simulink model "SF035A_DampgPahFwl"  (R2013b)
settings: Solver=FixedStepDiscrete  SolverMode=SingleTasking  StartTime=0.0  StopTime=1  FixedStep=0.002  RelTol=1e-3
undefined symbols (not defined in the file): ARCHGLBPRM_2MILLISEC_SEC_F32, DampgPahFwlDampgCmdFwlOverLimDiagcFailStep, DampgPahFwlDampgCmdFwlOverLimDiagcPassStep, DampgPahFwlInertiaCmpCmdFwlOverLimDiagcFailStep, DampgPahFwlInertiaCmpCmdFwlOverLimDiagcPassStep, DMPGCMDREACHED_CNT_U08, MfgEnaSt1, NtcNr1, NtcSts1, sigbuilder_block, SigQlfr1, VBICCMDREACHED_CNT_U08
libraries: simulink x23, Fil x12, FixdToFloat x7, FloatToFixd x5, BilnrIntrpnCmnX x4, LnrIntrpn x3, NxtrLim x3, NxtrAbslt x2, NxtrSign x2, NxtrMax x1
(part 2 of 3)

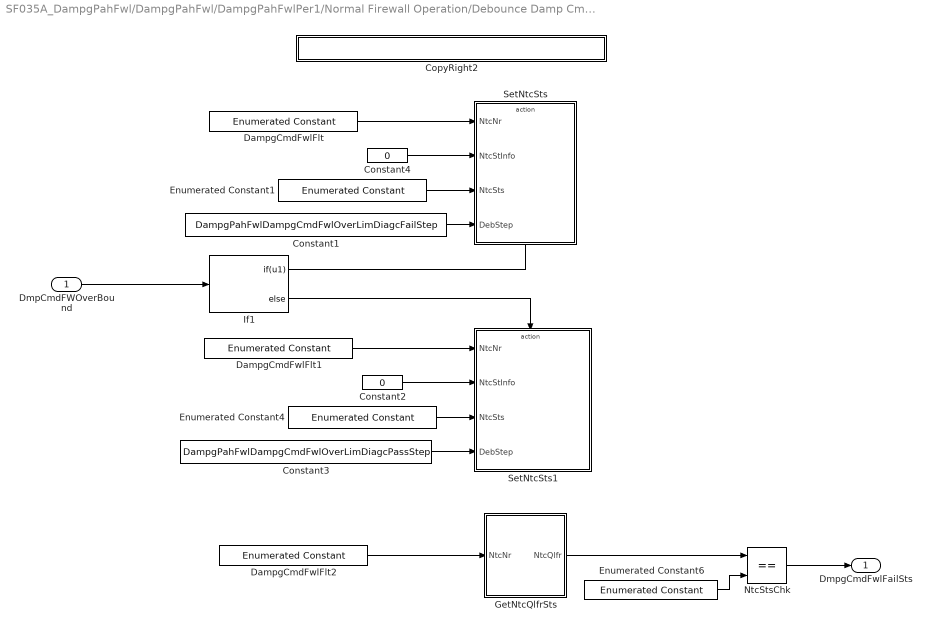
== system SF035A_DampgPahFwl/DampgPahFwl/DampgPahFwlPer1/Normal Firewall Operation/Debounce Damp Cmd Overboundary ==
  DmpCmdFWOverBound : Inport
  Constant1 : Constant  Value=DampgPahFwlDampgCmdFwlOverLimDiagcFailStep  OutDataTypeStr=uint16
  Constant2 : Constant  RequirementInfo={} %GIDa_55bfd7d4_70c1_4792_a0e0_29b38575031f  Value=0  OutDataTypeStr=uint8
      settings: AttributesFormatString=%<OutDataTypeStr>
  Constant3 : Constant  Value=DampgPahFwlDampgCmdFwlOverLimDiagcPassStep  OutDataTypeStr=uint16
  Constant4 : Constant  RequirementInfo={} %GIDa_7ee0dd85_1d59_46bb_85d2_699fcecf5629  Value=0  OutDataTypeStr=uint8
      settings: AttributesFormatString=%<OutDataTypeStr>
  CopyRight2 : Subsystem  Description=|  mask(Copyright Information){none=on}
      | Copyright info block.                                               
      |                                                                     
      | Place copyright information at the top of every subsystem in design.
      mask prompts: none "No parameters"
      mask help: Place copyright information at the top of every subsystem in design.
      mask Display:
      | NxtrConf = 'Nexteer Confidential';
      | 
      | sys = bdroot; %handle for the current model ("system")
      | first = get_param(sys,'Created');
      | first = first(end-3:end);  %year is last four digits
      | 
      | last = get_param(sys,'LastModifiedDate');
      | if isempty(last)
      |     last = datestr(now,'yyyy');
      | else
      |     last = last(end-3:end);
      | end
      | 
      | if strcmp(first,last)
      |     fprintf('%s -- Copyright %s Nexteer',NxtrConf,first)
      | else
      |     fprintf('%s -- %s%s- %s Nexteer',NxtrConf,char(169),first,last)
      | end
  DampgCmdFwlFlt : simulink/Sources/Enumerated Constant  OutDataTypeStr=Enum: NtcNr1  Value=NtcNr1.NTCNR_0X0D4  SampleTime=inf
  DampgCmdFwlFlt1 : simulink/Sources/Enumerated Constant  OutDataTypeStr=Enum: NtcNr1  Value=NtcNr1.NTCNR_0X0D4  SampleTime=inf
  "DampgCmdFwlFlt2 " : simulink/Sources/Enumerated Constant  OutDataTypeStr=Enum: NtcNr1  Value=NtcNr1.NTCNR_0X0D4  SampleTime=inf
  Enumerated Constant1 : simulink/Sources/Enumerated Constant  OutDataTypeStr=Enum: NtcSts1  Value=NtcSts1.NTCSTS_PREFAILD  SampleTime=inf
  Enumerated Constant4 : simulink/Sources/Enumerated Constant  OutDataTypeStr=Enum: NtcSts1  Value=NtcSts1.NTCSTS_PREPASSD  SampleTime=inf
  Enumerated Constant6 : simulink/Sources/Enumerated Constant  RequirementInfo={} %GIDa_97c32d1f_6dd1_433b_809d_2a860277b6b3  OutDataTypeStr=Enum: SigQlfr1  Value=SigQlfr1.SIGQLFR_FAILD  SampleTime=inf
  GetNtcQlfrSts : Subsystem  RequirementInfo={} %GIDa_0bc7a28c_a9ac_4638_a090_8c7002d6c785  TreatAsAtomicUnit=on  mask(GetNTC){}
      mask help: GetNTC library block
      settings: RTWSystemCode=Inline
  If1 : If  IfExpression=u1
  NtcStsChk : RelationalOperator  RequirementInfo={} %GIDa_d9fc4157_cb24_49cf_a4b6_ee40b9a9ec3d  Operator===  OutDataTypeStr=boolean
  SetNtcSts : Subsystem  mask(SetNTC){}
      mask help: SetNTC library block
  SetNtcSts1 : Subsystem  mask(SetNTC){}
      mask help: SetNTC library block
  DmpgCmdFwlFailSts : Outport
  wires:
  Enumerated Constant1/1 -> SetNtcSts/3(NtcSts)
  Constant1/1 -> SetNtcSts/4(DebStep)
  Constant4/1 -> SetNtcSts/2(NtcStInfo)
  Constant2/1 -> SetNtcSts1/2(NtcStInfo)
  Enumerated Constant4/1 -> SetNtcSts1/3(NtcSts)
  Constant3/1 -> SetNtcSts1/4(DebStep)
  Enumerated Constant6/1 -> NtcStsChk/2
  NtcStsChk/1 -> DmpgCmdFwlFailSts/1
  GetNtcQlfrSts/1(NtcQlfr) -> NtcStsChk/1
  DmpCmdFWOverBound/1 -> If1/1
  DampgCmdFwlFlt/1 -> SetNtcSts/1(NtcNr)
  DampgCmdFwlFlt1/1 -> SetNtcSts1/1(NtcNr)
  "DampgCmdFwlFlt2 "/1 -> GetNtcQlfrSts/1(NtcNr)
  If1/1 -> SetNtcSts/Action
  If1/2 -> SetNtcSts1/Action

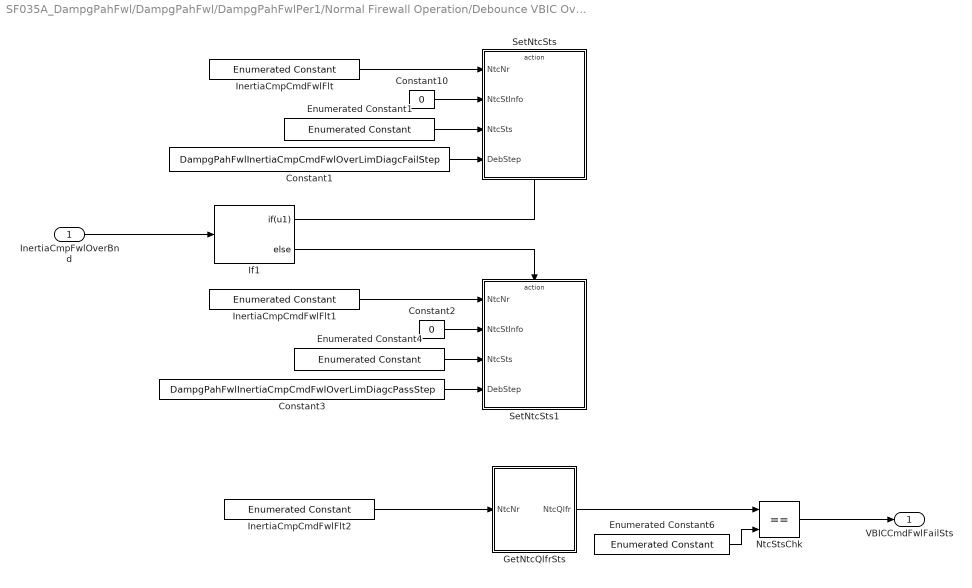
== system SF035A_DampgPahFwl/DampgPahFwl/DampgPahFwlPer1/Normal Firewall Operation/Debounce VBIC Overboundary ==
  InertiaCmpFwlOverBnd : Inport
  Constant1 : Constant  Value=DampgPahFwlInertiaCmpCmdFwlOverLimDiagcFailStep  OutDataTypeStr=uint16
  Constant10 : Constant  Value=0
  Constant2 : Constant  Value=0
  Constant3 : Constant  Value=DampgPahFwlInertiaCmpCmdFwlOverLimDiagcPassStep  OutDataTypeStr=uint16
  Enumerated Constant1 : simulink/Sources/Enumerated Constant  OutDataTypeStr=Enum: NtcSts1  Value=NtcSts1.NTCSTS_PREFAILD  SampleTime=inf
  Enumerated Constant4 : simulink/Sources/Enumerated Constant  OutDataTypeStr=Enum: NtcSts1  Value=NtcSts1.NTCSTS_PREPASSD  SampleTime=inf
  Enumerated Constant6 : simulink/Sources/Enumerated Constant  RequirementInfo={} %GIDa_dc6df379_4f99_41ef_b6ae_731f9d8bc089  OutDataTypeStr=Enum: SigQlfr1  Value=SigQlfr1.SIGQLFR_FAILD  SampleTime=inf
  GetNtcQlfrSts : Subsystem  RequirementInfo={} %GIDa_a84cbcff_9679_4c8a_9540_236060a0f7ef  TreatAsAtomicUnit=on  mask(GetNTC){}
      mask help: GetNTC library block
      settings: RTWSystemCode=Inline
  If1 : If  IfExpression=u1
  InertiaCmpCmdFwlFlt : simulink/Sources/Enumerated Constant  OutDataTypeStr=Enum: NtcNr1  Value=NtcNr1.NTCNR_0X0D5  SampleTime=inf
  InertiaCmpCmdFwlFlt1 : simulink/Sources/Enumerated Constant  OutDataTypeStr=Enum: NtcNr1  Value=NtcNr1.NTCNR_0X0D5  SampleTime=inf
  InertiaCmpCmdFwlFlt2 : simulink/Sources/Enumerated Constant  OutDataTypeStr=Enum: NtcNr1  Value=NtcNr1.NTCNR_0X0D5  SampleTime=inf
  NtcStsChk : RelationalOperator  RequirementInfo={} %GIDa_3e5098cd_7e63_4820_8b9b_1c92b23f34a0  Operator===  OutDataTypeStr=boolean
  SetNtcSts : Subsystem  mask(SetNTC){}
      mask help: SetNTC library block
  SetNtcSts1 : Subsystem  mask(SetNTC){}
      mask help: SetNTC library block
  VBICCmdFwlFailSts : Outport
  wires:
  Enumerated Constant1/1 -> SetNtcSts/3(NtcSts)
  Constant1/1 -> SetNtcSts/4(DebStep)
  Constant10/1 -> SetNtcSts/2(NtcStInfo)
  Constant2/1 -> SetNtcSts1/2(NtcStInfo)
  Enumerated Constant4/1 -> SetNtcSts1/3(NtcSts)
  Constant3/1 -> SetNtcSts1/4(DebStep)
  Enumerated Constant6/1 -> NtcStsChk/2
  NtcStsChk/1 -> VBICCmdFwlFailSts/1
  GetNtcQlfrSts/1(NtcQlfr) -> NtcStsChk/1
  InertiaCmpFwlOverBnd/1 -> If1/1
  InertiaCmpCmdFwlFlt/1 -> SetNtcSts/1(NtcNr)
  InertiaCmpCmdFwlFlt1/1 -> SetNtcSts1/1(NtcNr)
  InertiaCmpCmdFwlFlt2/1 -> GetNtcQlfrSts/1(NtcNr)
  If1/1 -> SetNtcSts/Action
  If1/2 -> SetNtcSts1/Action

== system SF035A_DampgPahFwl/DampgPahFwl/DampgPahFwlPer1/Normal Firewall Operation/Default Damping ==
  DefltDamp : Inport
  Action Port : ActionPort  ActionType=then
  Constant1 : Constant  Value=true  OutDataTypeStr=boolean
      settings: AttributesFormatString=%<OutDataTypeStr>
  Constant3 : Constant  Value=0  OutDataTypeStr=single
      settings: AttributesFormatString=%<OutDataTypeStr>
  CopyRight2 : Subsystem  Description=|  mask(Copyright Information){none=on}
      | Copyright info block.                                               
      |                                                                     
      | Place copyright information at the top of every subsystem in design.
      mask prompts: none "No parameters"
      mask help: Place copyright information at the top of every subsystem in design.
      mask Display:
      | NxtrConf = 'Nexteer Confidential';
      | 
      | sys = bdroot; %handle for the current model ("system")
      | first = get_param(sys,'Created');
      | first = first(end-3:end);  %year is last four digits
      | 
      | last = get_param(sys,'LastModifiedDate');
      | if isempty(last)
      |     last = datestr(now,'yyyy');
      | else
      |     last = last(end-3:end);
      | end
      | 
      | if strcmp(first,last)
      |     fprintf('%s -- Copyright %s Nexteer',NxtrConf,first)
      | else
      |     fprintf('%s -- %s%s- %s Nexteer',NxtrConf,char(169),first,last)
      | end
  DampgCmd : Outport
  DampgFwlActvRaw : Outport  Port=2
  DampgReducedPrfmnc : Outport  Port=3
  wires:
  Constant1/1 -> DampgReducedPrfmnc/1
  Constant3/1 -> DampgFwlActvRaw/1
  DefltDamp/1 -> DampgCmd/1

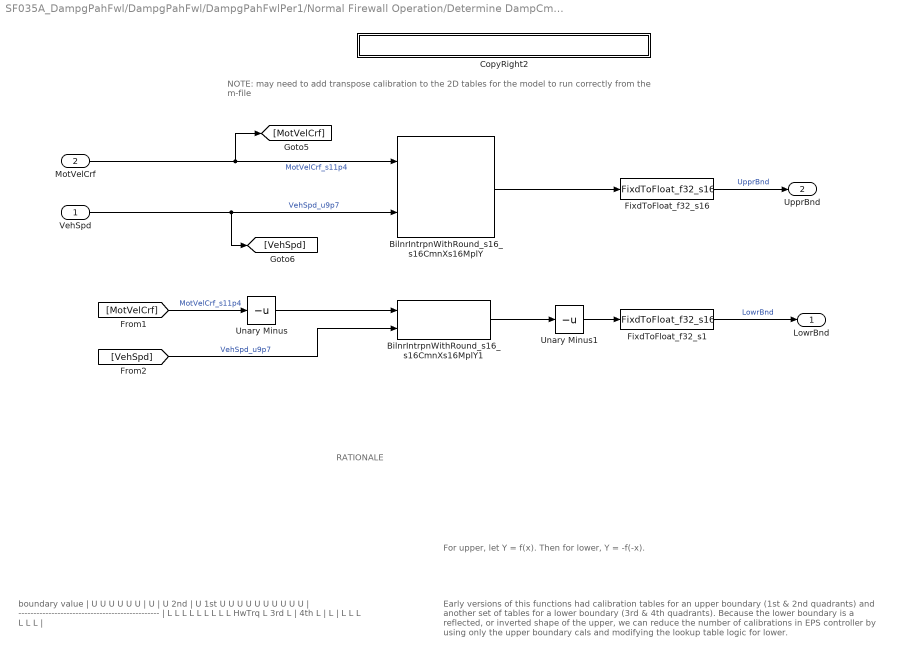
== system SF035A_DampgPahFwl/DampgPahFwl/DampgPahFwlPer1/Normal Firewall Operation/Determine DampCmd Boundaries ==
  note: boundary value
      |                    |       U U U U U U
      |                    |     U
      |                    |   U
      |       2nd          | U       1st
      |                    U
      |  U U U U U U U U U |
      | -----------------------------------------------
      |                    | L L L L L L L L L    HwTrq
      |                    L
      |       3rd        L |         4th
      |                L   |
      |              L     |
      |  L L L L L L       |
  note: RATIONALE
  note: Early versions of this functions had calibration tables for an upper boundary (1st & 2nd quadrants)
      | and another set of tables for a lower boundary (3rd & 4th quadrants).  Because the lower boundary
      | is a reflected, or inverted shape of the upper, we can reduce the number of calibrations in EPS
      | controller by using only the upper boundary cals and modifying the lookup table logic for lower.
  note: For upper, let Y = f(x). Then for lower, Y = -f(-x).
  note: NOTE: may need to add transpose calibration to the 2D tables for the model to run correctly from the m-file
  VehSpd : Inport
  MotVelCrf : Inport  Port=2
  BilnrIntrpnWithRound_s16_s16CmnXs16MplY : BilnrIntrpnCmnX/BilnrIntrpnWithRound_s16_s16CmnXs16MplY  XTbl=DampgPahFwlDampgCmdUpprLimX  MplYTbl=DampgPahFwlDampgCmdUpprLimY  BilnrSelnTbl=DampgPahFwlVehSpd
      settings: AttributesFormatString=Bilnr ( s16CmnX , s16MplY )
  BilnrIntrpnWithRound_s16_s16CmnXs16MplY1 : BilnrIntrpnCmnX/BilnrIntrpnWithRound_s16_s16CmnXs16MplY  XTbl=DampgPahFwlDampgCmdUpprLimX  MplYTbl=DampgPahFwlDampgCmdUpprLimY  BilnrSelnTbl=DampgPahFwlVehSpd
      settings: AttributesFormatString=Bilnr ( s16CmnX , s16MplY )
  CopyRight2 : Subsystem  Description=|  mask(Copyright Information){none=on}
      | Copyright info block.                                               
      |                                                                     
      | Place copyright information at the top of every subsystem in design.
      mask prompts: none "No parameters"
      mask help: Place copyright information at the top of every subsystem in design.
      mask Display:
      | NxtrConf = 'Nexteer Confidential';
      | 
      | sys = bdroot; %handle for the current model ("system")
      | first = get_param(sys,'Created');
      | first = first(end-3:end);  %year is last four digits
      | 
      | last = get_param(sys,'LastModifiedDate');
      | if isempty(last)
      |     last = datestr(now,'yyyy');
      | else
      |     last = last(end-3:end);
      | end
      | 
      | if strcmp(first,last)
      |     fprintf('%s -- Copyright %s Nexteer',NxtrConf,first)
      | else
      |     fprintf('%s -- %s%s- %s Nexteer',NxtrConf,char(169),first,last)
      | end
  FixdToFloat_f32_s1 : FixdToFloat/FixdToFloat_f32_s16  Param1=8
  FixdToFloat_f32_s16 : FixdToFloat/FixdToFloat_f32_s16  Param1=8
  Unary Minus : UnaryMinus
  Unary Minus1 : UnaryMinus
  LowrBnd : Outport
  UpprBnd : Outport  Port=2
  wires:
  FixdToFloat_f32_s16/1 -> UpprBnd/1  "UpprBnd"
  [MotVelCrf] -> Unary Minus/1  "MotVelCrf_s11p4"
  Unary Minus1/1 -> FixdToFloat_f32_s1/1
  MotVelCrf/1 -> BilnrIntrpnWithRound_s16_s16CmnXs16MplY/1, [MotVelCrf]  "MotVelCrf_s11p4"
  VehSpd/1 -> BilnrIntrpnWithRound_s16_s16CmnXs16MplY/2, [VehSpd]  "VehSpd_u9p7"
  BilnrIntrpnWithRound_s16_s16CmnXs16MplY/1 -> FixdToFloat_f32_s16/1
  FixdToFloat_f32_s1/1 -> LowrBnd/1  "LowrBnd"
  BilnrIntrpnWithRound_s16_s16CmnXs16MplY1/1 -> Unary Minus1/1
  Unary Minus/1 -> BilnrIntrpnWithRound_s16_s16CmnXs16MplY1/1
  [VehSpd] -> BilnrIntrpnWithRound_s16_s16CmnXs16MplY1/2  "VehSpd_u9p7"

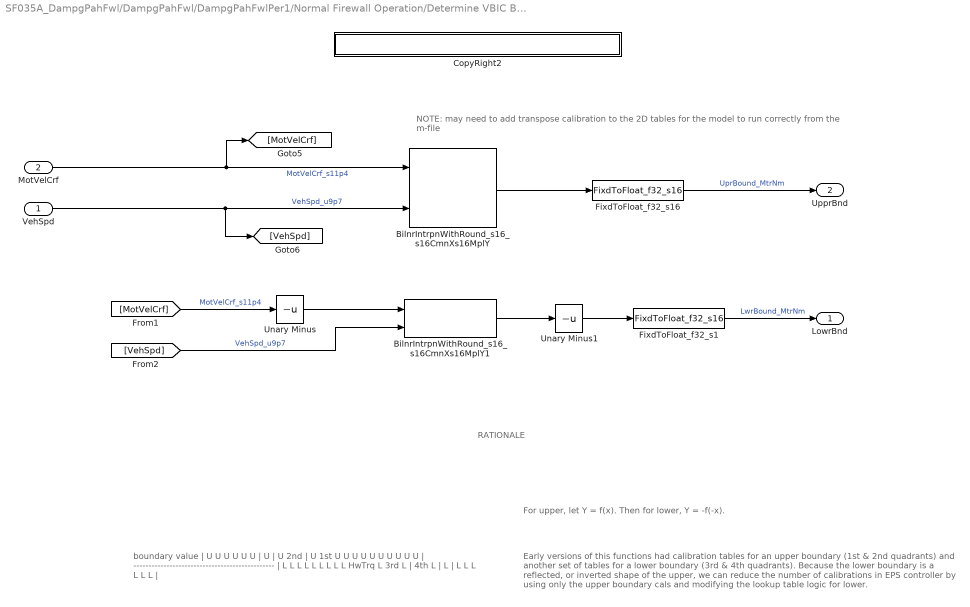
== system SF035A_DampgPahFwl/DampgPahFwl/DampgPahFwlPer1/Normal Firewall Operation/Determine VBIC Boundaries ==
  note: NOTE: may need to add transpose calibration to the 2D tables for the model to run correctly from the m-file
  note: boundary value
      |                    |       U U U U U U
      |                    |     U
      |                    |   U
      |       2nd          | U       1st
      |                    U
      |  U U U U U U U U U |
      | -----------------------------------------------
      |                    | L L L L L L L L L    HwTrq
      |                    L
      |       3rd        L |         4th
      |                L   |
      |              L     |
      |  L L L L L L       |
  note: RATIONALE
  note: Early versions of this functions had calibration tables for an upper boundary (1st & 2nd quadrants)
      | and another set of tables for a lower boundary (3rd & 4th quadrants).  Because the lower boundary
      | is a reflected, or inverted shape of the upper, we can reduce the number of calibrations in EPS
      | controller by using only the upper boundary cals and modifying the lookup table logic for lower.
  note: For upper, let Y = f(x). Then for lower, Y = -f(-x).
  VehSpd : Inport
  "MotVelCrf " : Inport  Port=2
  BilnrIntrpnWithRound_s16_s16CmnXs16MplY : BilnrIntrpnCmnX/BilnrIntrpnWithRound_s16_s16CmnXs16MplY  XTbl=DampgPahFwlInertiaCmpUpprLimX  MplYTbl=DampgPahFwlInertiaCmpUpprLimY  BilnrSelnTbl=DampgPahFwlVehSpd
      settings: AttributesFormatString=Bilnr ( s16CmnX , s16MplY )
  BilnrIntrpnWithRound_s16_s16CmnXs16MplY1 : BilnrIntrpnCmnX/BilnrIntrpnWithRound_s16_s16CmnXs16MplY  XTbl=DampgPahFwlInertiaCmpUpprLimX  MplYTbl=DampgPahFwlInertiaCmpUpprLimY  BilnrSelnTbl=DampgPahFwlVehSpd
      settings: AttributesFormatString=Bilnr ( s16CmnX , s16MplY )
  CopyRight2 : Subsystem  Description=|  mask(Copyright Information){none=on}
      | Copyright info block.                                               
      |                                                                     
      | Place copyright information at the top of every subsystem in design.
      mask prompts: none "No parameters"
      mask help: Place copyright information at the top of every subsystem in design.
      mask Display:
      | NxtrConf = 'Nexteer Confidential';
      | 
      | sys = bdroot; %handle for the current model ("system")
      | first = get_param(sys,'Created');
      | first = first(end-3:end);  %year is last four digits
      | 
      | last = get_param(sys,'LastModifiedDate');
      | if isempty(last)
      |     last = datestr(now,'yyyy');
      | else
      |     last = last(end-3:end);
      | end
      | 
      | if strcmp(first,last)
      |     fprintf('%s -- Copyright %s Nexteer',NxtrConf,first)
      | else
      |     fprintf('%s -- %s%s- %s Nexteer',NxtrConf,char(169),first,last)
      | end
  FixdToFloat_f32_s1 : FixdToFloat/FixdToFloat_f32_s16  Param1=8
  FixdToFloat_f32_s16 : FixdToFloat/FixdToFloat_f32_s16  Param1=8
  Unary Minus : UnaryMinus
  Unary Minus1 : UnaryMinus
  LowrBnd : Outport
  UpprBnd : Outport  Port=2
  wires:
  BilnrIntrpnWithRound_s16_s16CmnXs16MplY/1 -> FixdToFloat_f32_s16/1
  BilnrIntrpnWithRound_s16_s16CmnXs16MplY1/1 -> Unary Minus1/1
  [MotVelCrf] -> Unary Minus/1  "MotVelCrf_s11p4"
  Unary Minus1/1 -> FixdToFloat_f32_s1/1
  FixdToFloat_f32_s16/1 -> UpprBnd/1  "UprBound_MtrNm"
  FixdToFloat_f32_s1/1 -> LowrBnd/1  "LwrBound_MtrNm"
  "MotVelCrf "/1 -> BilnrIntrpnWithRound_s16_s16CmnXs16MplY/1, [MotVelCrf]  "MotVelCrf_s11p4"
  VehSpd/1 -> [VehSpd], BilnrIntrpnWithRound_s16_s16CmnXs16MplY/2  "VehSpd_u9p7"
  Unary Minus/1 -> BilnrIntrpnWithRound_s16_s16CmnXs16MplY1/1
  [VehSpd] -> BilnrIntrpnWithRound_s16_s16CmnXs16MplY1/2  "VehSpd_u9p7"

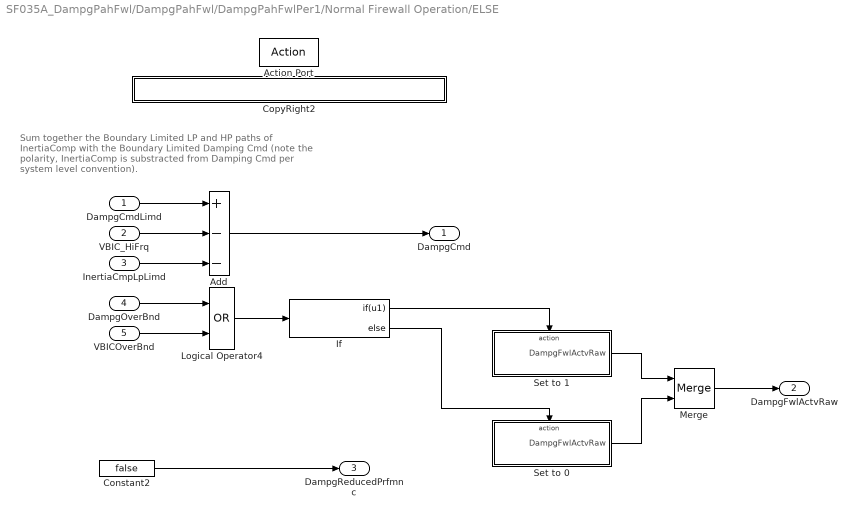
== system SF035A_DampgPahFwl/DampgPahFwl/DampgPahFwlPer1/Normal Firewall Operation/ELSE ==
  note: Sum together the Boundary Limited LP and HP paths of
      | InertiaComp with the Boundary Limited Damping Cmd
      | (note the polarity, InertiaComp is substracted from
      | Damping Cmd per system level convention).
  DampgCmdLimd : Inport
  VBIC_HiFrq : Inport  Port=2
  InertiaCmpLpLimd : Inport  Port=3
  DampgOverBnd : Inport  Port=4
  VBICOverBnd : Inport  Port=5
  Action Port : ActionPort  ActionType=else
  Add : Sum  Inputs=+--
  Constant2 : Constant  Value=false  OutDataTypeStr=boolean
      settings: AttributesFormatString=%<OutDataTypeStr>
  CopyRight2 : Subsystem  Description=|  mask(Copyright Information){none=on}
      | Copyright info block.                                               
      |                                                                     
      | Place copyright information at the top of every subsystem in design.
      mask prompts: none "No parameters"
      mask help: Place copyright information at the top of every subsystem in design.
      mask Display:
      | NxtrConf = 'Nexteer Confidential';
      | 
      | sys = bdroot; %handle for the current model ("system")
      | first = get_param(sys,'Created');
      | first = first(end-3:end);  %year is last four digits
      | 
      | last = get_param(sys,'LastModifiedDate');
      | if isempty(last)
      |     last = datestr(now,'yyyy');
      | else
      |     last = last(end-3:end);
      | end
      | 
      | if strcmp(first,last)
      |     fprintf('%s -- Copyright %s Nexteer',NxtrConf,first)
      | else
      |     fprintf('%s -- %s%s- %s Nexteer',NxtrConf,char(169),first,last)
      | end
  If : If  IfExpression=u1
  Logical Operator4 : Logic  Operator=OR  AllPortsSameDT=off  OutDataTypeStr=boolean
  Merge : Merge
  Set to 0 : Subsystem  TreatAsAtomicUnit=on
  Set to 1 : Subsystem  TreatAsAtomicUnit=on
  DampgCmd : Outport
  DampgFwlActvRaw : Outport  Port=2
  DampgReducedPrfmnc : Outport  Port=3
  wires:
  Add/1 -> DampgCmd/1
  Merge/1 -> DampgFwlActvRaw/1
  Constant2/1 -> DampgReducedPrfmnc/1
  DampgCmdLimd/1 -> Add/1
  InertiaCmpLpLimd/1 -> Add/3
  VBIC_HiFrq/1 -> Add/2
  Logical Operator4/1 -> If/1
  DampgOverBnd/1 -> Logical Operator4/1
  VBICOverBnd/1 -> Logical Operator4/2
  If/1 -> Set to 1/Action
  If/2 -> Set to 0/Action
  Set to 1/1(DampgFwlActvRaw) -> Merge/1
  Set to 0/1(DampgFwlActvRaw) -> Merge/2

== system SF035A_DampgPahFwl/DampgPahFwl/DampgPahFwlPer1/Normal Firewall Operation/FWActive LP Filter ==
  FwlActvRaw : Inport
  CopyRight2 : Subsystem  Description=|  mask(Copyright Information){none=on}
      | Copyright info block.                                               
      |                                                                     
      | Place copyright information at the top of every subsystem in design.
      mask prompts: none "No parameters"
      mask help: Place copyright information at the top of every subsystem in design.
      mask Display:
      | NxtrConf = 'Nexteer Confidential';
      | 
      | sys = bdroot; %handle for the current model ("system")
      | first = get_param(sys,'Created');
      | first = first(end-3:end);  %year is last four digits
      | 
      | last = get_param(sys,'LastModifiedDate');
      | if isempty(last)
      |     last = datestr(now,'yyyy');
      | else
      |     last = last(end-3:end);
      | end
      | 
      | if strcmp(first,last)
      |     fprintf('%s -- Copyright %s Nexteer',NxtrConf,first)
      | else
      |     fprintf('%s -- %s%s- %s Nexteer',NxtrConf,char(169),first,last)
      | end
  FilLpUpdOutp : Fil/FilLpUpdOutp  StVar=FwlActvLpFil
      settings: AttributesFormatString=StVar: %<StVar>
  FwlActvLpFil : Outport
  wires:
  FwlActvRaw/1 -> FilLpUpdOutp/1
  FilLpUpdOutp/1 -> FwlActvLpFil/1

== system SF035A_DampgPahFwl/DampgPahFwl/DampgPahFwlPer1/Normal Firewall Operation/Low Pass Filter DmpCmd Boundaries ==
  LowrBnd : Inport
  UpprBnd : Inport  Port=2
  CopyRight2 : Subsystem  Description=|  mask(Copyright Information){none=on}
      | Copyright info block.                                               
      |                                                                     
      | Place copyright information at the top of every subsystem in design.
      mask prompts: none "No parameters"
      mask help: Place copyright information at the top of every subsystem in design.
      mask Display:
      | NxtrConf = 'Nexteer Confidential';
      | 
      | sys = bdroot; %handle for the current model ("system")
      | first = get_param(sys,'Created');
      | first = first(end-3:end);  %year is last four digits
      | 
      | last = get_param(sys,'LastModifiedDate');
      | if isempty(last)
      |     last = datestr(now,'yyyy');
      | else
      |     last = last(end-3:end);
      | end
      | 
      | if strcmp(first,last)
      |     fprintf('%s -- Copyright %s Nexteer',NxtrConf,first)
      | else
      |     fprintf('%s -- %s%s- %s Nexteer',NxtrConf,char(169),first,last)
      | end
  FilLpUpdOutp : Fil/FilLpUpdOutp  StVar=DampgCmdLpFilLowrLim
      settings: AttributesFormatString=StVar: %<StVar>
  FilLpUpdOutp1 : Fil/FilLpUpdOutp  StVar=DampgCmdLpFilUpprLim
      settings: AttributesFormatString=StVar: %<StVar>
  LowrBndLpFil : Outport
  UpprBndLpFil : Outport  Port=2
  wires:
  LowrBnd/1 -> FilLpUpdOutp/1
  FilLpUpdOutp/1 -> LowrBndLpFil/1
  FilLpUpdOutp1/1 -> UpprBndLpFil/1
  UpprBnd/1 -> FilLpUpdOutp1/1

== system SF035A_DampgPahFwl/DampgPahFwl/DampgPahFwlPer1/Normal Firewall Operation/Low Pass Filter VBIC Boundaries ==
  LowrBnd : Inport
  UpprBnd : Inport  Port=2
  CopyRight2 : Subsystem  Description=|  mask(Copyright Information){none=on}
      | Copyright info block.                                               
      |                                                                     
      | Place copyright information at the top of every subsystem in design.
      mask prompts: none "No parameters"
      mask help: Place copyright information at the top of every subsystem in design.
      mask Display:
      | NxtrConf = 'Nexteer Confidential';
      | 
      | sys = bdroot; %handle for the current model ("system")
      | first = get_param(sys,'Created');
      | first = first(end-3:end);  %year is last four digits
      | 
      | last = get_param(sys,'LastModifiedDate');
      | if isempty(last)
      |     last = datestr(now,'yyyy');
      | else
      |     last = last(end-3:end);
      | end
      | 
      | if strcmp(first,last)
      |     fprintf('%s -- Copyright %s Nexteer',NxtrConf,first)
      | else
      |     fprintf('%s -- %s%s- %s Nexteer',NxtrConf,char(169),first,last)
      | end
  FilLpUpdOutp : Fil/FilLpUpdOutp  StVar=InertiaCmpLpFilLowrLim
      settings: AttributesFormatString=StVar: %<StVar>
  FilLpUpdOutp1 : Fil/FilLpUpdOutp  StVar=InertiaCmpLpFilUpprLim
      settings: AttributesFormatString=StVar: %<StVar>
  LowrBndLpFil : Outport
  UpprBndLpFil : Outport  Port=2
  wires:
  FilLpUpdOutp/1 -> LowrBndLpFil/1
  LowrBnd/1 -> FilLpUpdOutp/1
  UpprBnd/1 -> FilLpUpdOutp1/1
  FilLpUpdOutp1/1 -> UpprBndLpFil/1

== system SF035A_DampgPahFwl/DampgPahFwl/DampgPahFwlPer1/Normal Firewall Operation/Set_Faults ==
  note: NEXTEER TROUBLE CODE
      | Number  TYPE   Name
      |
      |  0x0C5      F3      NTCNumber.NTC_Num_DampingFWReached
  DampgFwlReached : Inport  RequirementInfo={} %GIDa_02747d93_2b4d_4ff6_94cd_b92274162cc5
  VBICFwlReached : Inport  RequirementInfo={} %GIDa_4a00ea3a_b728_4ae4_97f3_c4b3e76466bb  Port=2
  CopyRight2 : Subsystem  Description=|  mask(Copyright Information){none=on}
      | Copyright info block.                                               
      |                                                                     
      | Place copyright information at the top of every subsystem in design.
      mask prompts: none "No parameters"
      mask help: Place copyright information at the top of every subsystem in design.
      mask Display:
      | NxtrConf = 'Nexteer Confidential';
      | 
      | sys = bdroot; %handle for the current model ("system")
      | first = get_param(sys,'Created');
      | first = first(end-3:end);  %year is last four digits
      | 
      | last = get_param(sys,'LastModifiedDate');
      | if isempty(last)
      |     last = datestr(now,'yyyy');
      | else
      |     last = last(end-3:end);
      | end
      | 
      | if strcmp(first,last)
      |     fprintf('%s -- Copyright %s Nexteer',NxtrConf,first)
      | else
      |     fprintf('%s -- %s%s- %s Nexteer',NxtrConf,char(169),first,last)
      | end
  If : If  IfExpression=u1  ShowElse=off
  Logical Operator : Logic  Operator=OR  AllPortsSameDT=off  OutDataTypeStr=boolean
  Set NtcDmpgFwlReached : Subsystem  TreatAsAtomicUnit=on
  wires:
  Logical Operator/1 -> If/1
  DampgFwlReached/1 -> Set NtcDmpgFwlReached/1(DampgFwlReached), Logical Operator/1
  VBICFwlReached/1 -> Set NtcDmpgFwlReached/2(VBICFwlReached), Logical Operator/2
  If/1 -> Set NtcDmpgFwlReached/Action

== system SF035A_DampgPahFwl/DampgPahFwl/DampgPahFwlInit1/SetNtcSts/SetNtcSts/CopyRight2 ==

== system SF035A_DampgPahFwl/DampgPahFwl/DampgPahFwlInit1/SetNtcSts1/SetNtcSts/CopyRight2 ==

== system SF035A_DampgPahFwl/DampgPahFwl/DampgPahFwlInit1/SetNtcSts2/SetNtcSts/CopyRight2 ==

== system SF035A_DampgPahFwl/DampgPahFwl/DampgPahFwlPer1/Normal Firewall Operation/Debounce Damp Cmd Overboundary/CopyRight2 ==

== system SF035A_DampgPahFwl/DampgPahFwl/DampgPahFwlPer1/Normal Firewall Operation/Debounce Damp Cmd Overboundary/GetNtcQlfrSts ==
  NtcNr : Inport
  CopyRight2 : Subsystem  Description=|  mask(Copyright Information){none=on}
      | Copyright info block.                                               
      |                                                                     
      | Place copyright information at the top of every subsystem in design.
      mask prompts: none "No parameters"
      mask help: Place copyright information at the top of every subsystem in design.
      mask Display:
      | NxtrConf = 'Nexteer Confidential';
      | 
      | sys = bdroot; %handle for the current model ("system")
      | first = get_param(sys,'Created');
      | first = first(end-3:end);  %year is last four digits
      | 
      | last = get_param(sys,'LastModifiedDate');
      | if isempty(last)
      |     last = datestr(now,'yyyy');
      | else
      |     last = last(end-3:end);
      | end
      | 
      | if strcmp(first,last)
      |     fprintf('%s -- Copyright %s Nexteer',NxtrConf,first)
      | else
      |     fprintf('%s -- %s%s- %s Nexteer',NxtrConf,char(169),first,last)
      | end
  Data Store Read : DataStoreRead  DataStoreName=Ntc0X0D4Qlfr
  Terminator : Terminator
  NtcQlfr : Outport
  wires:
  Data Store Read/1 -> NtcQlfr/1
  NtcNr/1 -> Terminator/1

== system SF035A_DampgPahFwl/DampgPahFwl/DampgPahFwlPer1/Normal Firewall Operation/Debounce Damp Cmd Overboundary/SetNtcSts ==
  NtcNr : Inport
  NtcStInfo : Inport  Port=2
  NtcSts : Inport  Port=3
  DebStep : Inport  Port=4
  CallDiagMgr : ActionPort  ActionType=then
  SetNtcSts : Subsystem  RequirementInfo={} %GIDa_af317633_e57a_401e_bbe6_d81ec8268150  TreatAsAtomicUnit=on
      settings: RTWSystemCode=Inline
  wires:
  NtcStInfo/1 -> SetNtcSts/2(NtcStInfo)
  DebStep/1 -> SetNtcSts/4(DebStep)
  NtcSts/1 -> SetNtcSts/3(NtcSts)
  NtcNr/1 -> SetNtcSts/1(NtcNr)  "NtcNr"

== system SF035A_DampgPahFwl/DampgPahFwl/DampgPahFwlPer1/Normal Firewall Operation/Debounce Damp Cmd Overboundary/SetNtcSts1 ==
  NtcNr : Inport
  NtcStInfo : Inport  Port=2
  NtcSts : Inport  Port=3
  DebStep : Inport  Port=4
  CallDiagMgr : ActionPort  ActionType=else
  SetNtcSts : Subsystem  RequirementInfo={} %GIDa_25cef4a2_5ef1_4a8e_bc54_aa7dce90260d  TreatAsAtomicUnit=on
      settings: RTWSystemCode=Inline
  wires:
  NtcNr/1 -> SetNtcSts/1(NtcNr)  "NtcNr"
  NtcSts/1 -> SetNtcSts/3(NtcSts)
  DebStep/1 -> SetNtcSts/4(DebStep)
  NtcStInfo/1 -> SetNtcSts/2(NtcStInfo)

== system SF035A_DampgPahFwl/DampgPahFwl/DampgPahFwlPer1/Normal Firewall Operation/Debounce VBIC Overboundary/GetNtcQlfrSts ==
  NtcNr : Inport
  CopyRight2 : Subsystem  Description=|  mask(Copyright Information){none=on}
      | Copyright info block.                                               
      |                                                                     
      | Place copyright information at the top of every subsystem in design.
      mask prompts: none "No parameters"
      mask help: Place copyright information at the top of every subsystem in design.
      mask Display:
      | NxtrConf = 'Nexteer Confidential';
      | 
      | sys = bdroot; %handle for the current model ("system")
      | first = get_param(sys,'Created');
      | first = first(end-3:end);  %year is last four digits
      | 
      | last = get_param(sys,'LastModifiedDate');
      | if isempty(last)
      |     last = datestr(now,'yyyy');
      | else
      |     last = last(end-3:end);
      | end
      | 
      | if strcmp(first,last)
      |     fprintf('%s -- Copyright %s Nexteer',NxtrConf,first)
      | else
      |     fprintf('%s -- %s%s- %s Nexteer',NxtrConf,char(169),first,last)
      | end
  Data Store Read : DataStoreRead  DataStoreName=Ntc0X0D5Qlfr
  Terminator : Terminator
  NtcQlfr : Outport
  wires:
  Data Store Read/1 -> NtcQlfr/1
  NtcNr/1 -> Terminator/1

== system SF035A_DampgPahFwl/DampgPahFwl/DampgPahFwlPer1/Normal Firewall Operation/Debounce VBIC Overboundary/SetNtcSts ==
  NtcNr : Inport
  NtcStInfo : Inport  Port=2
  NtcSts : Inport  Port=3
  DebStep : Inport  Port=4
  CallDiagMgr : ActionPort  ActionType=then
  SetNtcSts : Subsystem  RequirementInfo={} %GIDa_029f64ab_5558_46ef_a250_7274573eb945  TreatAsAtomicUnit=on
      settings: RTWSystemCode=Inline
  wires:
  NtcStInfo/1 -> SetNtcSts/2(NtcStInfo)
  DebStep/1 -> SetNtcSts/4(DebStep)
  NtcSts/1 -> SetNtcSts/3(NtcSts)
  NtcNr/1 -> SetNtcSts/1(NtcNr)  "NtcNr"

== system SF035A_DampgPahFwl/DampgPahFwl/DampgPahFwlPer1/Normal Firewall Operation/Debounce VBIC Overboundary/SetNtcSts1 ==
  NtcNr : Inport
  NtcStInfo : Inport  Port=2
  NtcSts : Inport  Port=3
  DebStep : Inport  Port=4
  CallDiagMgr : ActionPort  ActionType=else
  SetNtcSts : Subsystem  RequirementInfo={} %GIDa_4af8b83c_cb93_4090_a015_cd2ccf4b901b  TreatAsAtomicUnit=on
      settings: RTWSystemCode=Inline
  wires:
  NtcNr/1 -> SetNtcSts/1(NtcNr)  "NtcNr"
  NtcSts/1 -> SetNtcSts/3(NtcSts)
  DebStep/1 -> SetNtcSts/4(DebStep)
  NtcStInfo/1 -> SetNtcSts/2(NtcStInfo)

== system SF035A_DampgPahFwl/DampgPahFwl/DampgPahFwlPer1/Normal Firewall Operation/Default Damping/CopyRight2 ==

== system SF035A_DampgPahFwl/DampgPahFwl/DampgPahFwlPer1/Normal Firewall Operation/Determine DampCmd Boundaries/CopyRight2 ==

== system SF035A_DampgPahFwl/DampgPahFwl/DampgPahFwlPer1/Normal Firewall Operation/Determine VBIC Boundaries/CopyRight2 ==

== system SF035A_DampgPahFwl/DampgPahFwl/DampgPahFwlPer1/Normal Firewall Operation/ELSE/CopyRight2 ==

== system SF035A_DampgPahFwl/DampgPahFwl/DampgPahFwlPer1/Normal Firewall Operation/ELSE/Set to 0 ==
  Action Port : ActionPort  ActionType=else
  Constant : Constant  Value=0  OutDataTypeStr=single
      settings: AttributesFormatString=%<OutDataTypeStr>
  DampgFwlActvRaw : Outport
  wires:
  Constant/1 -> DampgFwlActvRaw/1

== system SF035A_DampgPahFwl/DampgPahFwl/DampgPahFwlPer1/Normal Firewall Operation/ELSE/Set to 1 ==
  Action Port : ActionPort  ActionType=then
  Constant : Constant  OutDataTypeStr=single
      settings: AttributesFormatString=%<OutDataTypeStr>
  DampgFwlActvRaw : Outport
  wires:
  Constant/1 -> DampgFwlActvRaw/1

== system SF035A_DampgPahFwl/DampgPahFwl/DampgPahFwlPer1/Normal Firewall Operation/FWActive LP Filter/CopyRight2 ==

== system SF035A_DampgPahFwl/DampgPahFwl/DampgPahFwlPer1/Normal Firewall Operation/Low Pass Filter DmpCmd Boundaries/CopyRight2 ==

== system SF035A_DampgPahFwl/DampgPahFwl/DampgPahFwlPer1/Normal Firewall Operation/Low Pass Filter VBIC Boundaries/CopyRight2 ==

== system SF035A_DampgPahFwl/DampgPahFwl/DampgPahFwlPer1/Normal Firewall Operation/Set_Faults/CopyRight2 ==

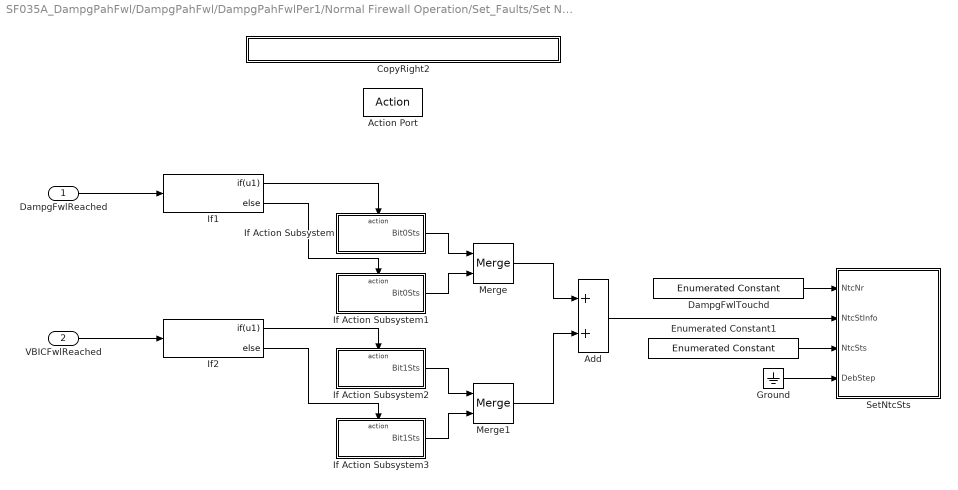
== system SF035A_DampgPahFwl/DampgPahFwl/DampgPahFwlPer1/Normal Firewall Operation/Set_Faults/Set NtcDmpgFwlReached ==
  DampgFwlReached : Inport
  VBICFwlReached : Inport  Port=2
  Action Port : ActionPort
  Add : Sum
  CopyRight2 : Subsystem  Description=|  mask(Copyright Information){none=on}
      | Copyright info block.                                               
      |                                                                     
      | Place copyright information at the top of every subsystem in design.
      mask prompts: none "No parameters"
      mask help: Place copyright information at the top of every subsystem in design.
      mask Display:
      | NxtrConf = 'Nexteer Confidential';
      | 
      | sys = bdroot; %handle for the current model ("system")
      | first = get_param(sys,'Created');
      | first = first(end-3:end);  %year is last four digits
      | 
      | last = get_param(sys,'LastModifiedDate');
      | if isempty(last)
      |     last = datestr(now,'yyyy');
      | else
      |     last = last(end-3:end);
      | end
      | 
      | if strcmp(first,last)
      |     fprintf('%s -- Copyright %s Nexteer',NxtrConf,first)
      | else
      |     fprintf('%s -- %s%s- %s Nexteer',NxtrConf,char(169),first,last)
      | end
  DampgFwlTouchd : simulink/Sources/Enumerated Constant  OutDataTypeStr=Enum: NtcNr1  Value=NtcNr1.NTCNR_0X0C5  SampleTime=inf
  Enumerated Constant1 : simulink/Sources/Enumerated Constant  OutDataTypeStr=Enum: NtcSts1  Value=NtcSts1.NTCSTS_FAILD  SampleTime=inf
  Ground : Ground
  If Action Subsystem : Subsystem  TreatAsAtomicUnit=on
  If Action Subsystem1 : Subsystem  TreatAsAtomicUnit=on
  If Action Subsystem2 : Subsystem  TreatAsAtomicUnit=on
  If Action Subsystem3 : Subsystem  TreatAsAtomicUnit=on
  If1 : If  IfExpression=u1
  If2 : If  IfExpression=u1
  Merge : Merge
  Merge1 : Merge
  SetNtcSts : Subsystem  mask(SetNTC){}
      mask help: SetNTC library block
  wires:
  DampgFwlTouchd/1 -> SetNtcSts/1(NtcNr)
  Enumerated Constant1/1 -> SetNtcSts/3(NtcSts)
  Ground/1 -> SetNtcSts/4(DebStep)
  DampgFwlReached/1 -> If1/1
  VBICFwlReached/1 -> If2/1
  If1/1 -> If Action Subsystem/Action
  If1/2 -> If Action Subsystem1/Action
  If2/1 -> If Action Subsystem2/Action
  If2/2 -> If Action Subsystem3/Action
  Add/1 -> SetNtcSts/2(NtcStInfo)
  If Action Subsystem/1(Bit0Sts) -> Merge/1
  If Action Subsystem1/1(Bit0Sts) -> Merge/2
  If Action Subsystem2/1(Bit1Sts) -> Merge1/1
  If Action Subsystem3/1(Bit1Sts) -> Merge1/2
  Merge/1 -> Add/1
  Merge1/1 -> Add/2

== system SF035A_DampgPahFwl/DampgPahFwl/DampgPahFwlPer1/Normal Firewall Operation/Debounce Damp Cmd Overboundary/GetNtcQlfrSts/CopyRight2 ==

== system SF035A_DampgPahFwl/DampgPahFwl/DampgPahFwlPer1/Normal Firewall Operation/Debounce Damp Cmd Overboundary/SetNtcSts/SetNtcSts ==
  note: Note:
      |
      | - "ISO Fault Debounce Design" Simulink block intent to use here for Simulation purpose only. Do not Code this block
  NtcNr : Inport
  NtcStInfo : Inport  Port=2
  NtcSts : Inport  Port=3
  DebStep : Inport  Port=4
  CopyRight2 : Subsystem  Description=|  mask(Copyright Information){none=on}
      | Copyright info block.                                               
      |                                                                     
      | Place copyright information at the top of every subsystem in design.
      mask prompts: none "No parameters"
      mask help: Place copyright information at the top of every subsystem in design.
      mask Display:
      | NxtrConf = 'Nexteer Confidential';
      | 
      | sys = bdroot; %handle for the current model ("system")
      | first = get_param(sys,'Created');
      | first = first(end-3:end);  %year is last four digits
      | 
      | last = get_param(sys,'LastModifiedDate');
      | if isempty(last)
      |     last = datestr(now,'yyyy');
      | else
      |     last = last(end-3:end);
      | end
      | 
      | if strcmp(first,last)
      |     fprintf('%s -- Copyright %s Nexteer',NxtrConf,first)
      | else
      |     fprintf('%s -- %s%s- %s Nexteer',NxtrConf,char(169),first,last)
      | end
  Data Store Write : DataStoreWrite  DataStoreName=Ntc0X0D4Qlfr
  Data Type Conversion : DataTypeConversion  OutDataTypeStr=Enum: SigQlfr1
  Ground : Ground
  ISO Fault Debounce Design : Stateflow chart  TreatAsAtomicUnit=on
      settings: AttributesFormatString=|
      | Simulation Purpose Only.
      | Do Not Code this block
      | Diagnostic Manager Owns this requirement
  Terminator : Terminator
  Terminator1 : Terminator
  wires:
  Ground/1 -> ISO Fault Debounce Design/3(SvcClr)
  ISO Fault Debounce Design/1(Qualifier) -> Data Type Conversion/1
  DebStep/1 -> ISO Fault Debounce Design/2(DebStep)
  NtcSts/1 -> ISO Fault Debounce Design/1(NtcSts)
  NtcNr/1 -> Terminator/1
  NtcStInfo/1 -> Terminator1/1
  Data Type Conversion/1 -> Data Store Write/1

== system SF035A_DampgPahFwl/DampgPahFwl/DampgPahFwlPer1/Normal Firewall Operation/Debounce Damp Cmd Overboundary/SetNtcSts1/SetNtcSts ==
  note: Note:
      |
      | - "ISO Fault Debounce Design" Simulink block intent to use here for Simulation purpose only. Do not Code this block
  NtcNr : Inport
  NtcStInfo : Inport  Port=2
  NtcSts : Inport  Port=3
  DebStep : Inport  Port=4
  CopyRight2 : Subsystem  Description=|  mask(Copyright Information){none=on}
      | Copyright info block.                                               
      |                                                                     
      | Place copyright information at the top of every subsystem in design.
      mask prompts: none "No parameters"
      mask help: Place copyright information at the top of every subsystem in design.
      mask Display:
      | NxtrConf = 'Nexteer Confidential';
      | 
      | sys = bdroot; %handle for the current model ("system")
      | first = get_param(sys,'Created');
      | first = first(end-3:end);  %year is last four digits
      | 
      | last = get_param(sys,'LastModifiedDate');
      | if isempty(last)
      |     last = datestr(now,'yyyy');
      | else
      |     last = last(end-3:end);
      | end
      | 
      | if strcmp(first,last)
      |     fprintf('%s -- Copyright %s Nexteer',NxtrConf,first)
      | else
      |     fprintf('%s -- %s%s- %s Nexteer',NxtrConf,char(169),first,last)
      | end
  Data Store Write : DataStoreWrite  DataStoreName=Ntc0X0D4Qlfr
  Data Type Conversion : DataTypeConversion  OutDataTypeStr=Enum: SigQlfr1
  Ground : Ground
  ISO Fault Debounce Design : Stateflow chart  TreatAsAtomicUnit=on
      settings: AttributesFormatString=|
      | Simulation Purpose Only.
      | Do Not Code this block
      | Diagnostic Manager Owns this requirement
  Terminator : Terminator
  Terminator1 : Terminator
  wires:
  NtcStInfo/1 -> Terminator1/1
  NtcNr/1 -> Terminator/1
  NtcSts/1 -> ISO Fault Debounce Design/1(NtcSts)
  DebStep/1 -> ISO Fault Debounce Design/2(DebStep)
  ISO Fault Debounce Design/1(Qualifier) -> Data Type Conversion/1
  Ground/1 -> ISO Fault Debounce Design/3(SvcClr)
  Data Type Conversion/1 -> Data Store Write/1

== system SF035A_DampgPahFwl/DampgPahFwl/DampgPahFwlPer1/Normal Firewall Operation/Debounce VBIC Overboundary/GetNtcQlfrSts/CopyRight2 ==

== system SF035A_DampgPahFwl/DampgPahFwl/DampgPahFwlPer1/Normal Firewall Operation/Debounce VBIC Overboundary/SetNtcSts/SetNtcSts ==
  note: Note:
      |
      | - "ISO Fault Debounce Design" Simulink block intent to use here for Simulation purpose only. Do not Code this block
  NtcNr : Inport
  NtcStInfo : Inport  Port=2
  NtcSts : Inport  Port=3
  DebStep : Inport  Port=4
  CopyRight2 : Subsystem  Description=|  mask(Copyright Information){none=on}
      | Copyright info block.                                               
      |                                                                     
      | Place copyright information at the top of every subsystem in design.
      mask prompts: none "No parameters"
      mask help: Place copyright information at the top of every subsystem in design.
      mask Display:
      | NxtrConf = 'Nexteer Confidential';
      | 
      | sys = bdroot; %handle for the current model ("system")
      | first = get_param(sys,'Created');
      | first = first(end-3:end);  %year is last four digits
      | 
      | last = get_param(sys,'LastModifiedDate');
      | if isempty(last)
      |     last = datestr(now,'yyyy');
      | else
      |     last = last(end-3:end);
      | end
      | 
      | if strcmp(first,last)
      |     fprintf('%s -- Copyright %s Nexteer',NxtrConf,first)
      | else
      |     fprintf('%s -- %s%s- %s Nexteer',NxtrConf,char(169),first,last)
      | end
  Data Store Write : DataStoreWrite  DataStoreName=Ntc0X0D5Qlfr
  Data Type Conversion : DataTypeConversion  OutDataTypeStr=Enum: SigQlfr1
  Ground : Ground
  ISO Fault Debounce Design : Stateflow chart  TreatAsAtomicUnit=on
      settings: AttributesFormatString=|
      | Simulation Purpose Only.
      | Do Not Code this block
      | Diagnostic Manager Owns this requirement
  Terminator : Terminator
  Terminator1 : Terminator
  wires:
  Ground/1 -> ISO Fault Debounce Design/3(SvcClr)
  ISO Fault Debounce Design/1(Qualifier) -> Data Type Conversion/1
  DebStep/1 -> ISO Fault Debounce Design/2(DebStep)
  NtcSts/1 -> ISO Fault Debounce Design/1(NtcSts)
  NtcNr/1 -> Terminator/1
  NtcStInfo/1 -> Terminator1/1
  Data Type Conversion/1 -> Data Store Write/1

== system SF035A_DampgPahFwl/DampgPahFwl/DampgPahFwlPer1/Normal Firewall Operation/Debounce VBIC Overboundary/SetNtcSts1/SetNtcSts ==
  note: Note:
      |
      | - "ISO Fault Debounce Design" Simulink block intent to use here for Simulation purpose only. Do not Code this block
  NtcNr : Inport
  NtcStInfo : Inport  Port=2
  NtcSts : Inport  Port=3
  DebStep : Inport  Port=4
  CopyRight2 : Subsystem  Description=|  mask(Copyright Information){none=on}
      | Copyright info block.                                               
      |                                                                     
      | Place copyright information at the top of every subsystem in design.
      mask prompts: none "No parameters"
      mask help: Place copyright information at the top of every subsystem in design.
      mask Display:
      | NxtrConf = 'Nexteer Confidential';
      | 
      | sys = bdroot; %handle for the current model ("system")
      | first = get_param(sys,'Created');
      | first = first(end-3:end);  %year is last four digits
      | 
      | last = get_param(sys,'LastModifiedDate');
      | if isempty(last)
      |     last = datestr(now,'yyyy');
      | else
      |     last = last(end-3:end);
      | end
      | 
      | if strcmp(first,last)
      |     fprintf('%s -- Copyright %s Nexteer',NxtrConf,first)
      | else
      |     fprintf('%s -- %s%s- %s Nexteer',NxtrConf,char(169),first,last)
      | end
  Data Store Write : DataStoreWrite  DataStoreName=Ntc0X0D5Qlfr
  Data Type Conversion : DataTypeConversion  OutDataTypeStr=Enum: SigQlfr1
  Ground : Ground
  ISO Fault Debounce Design : Stateflow chart  TreatAsAtomicUnit=on
      settings: AttributesFormatString=|
      | Simulation Purpose Only.
      | Do Not Code this block
      | Diagnostic Manager Owns this requirement
  Terminator : Terminator
  Terminator1 : Terminator
  wires:
  NtcStInfo/1 -> Terminator1/1
  NtcNr/1 -> Terminator/1
  NtcSts/1 -> ISO Fault Debounce Design/1(NtcSts)
  DebStep/1 -> ISO Fault Debounce Design/2(DebStep)
  ISO Fault Debounce Design/1(Qualifier) -> Data Type Conversion/1
  Ground/1 -> ISO Fault Debounce Design/3(SvcClr)
  Data Type Conversion/1 -> Data Store Write/1

== system SF035A_DampgPahFwl/DampgPahFwl/DampgPahFwlPer1/Normal Firewall Operation/Set_Faults/Set NtcDmpgFwlReached/CopyRight2 ==

== system SF035A_DampgPahFwl/DampgPahFwl/DampgPahFwlPer1/Normal Firewall Operation/Set_Faults/Set NtcDmpgFwlReached/If Action Subsystem ==
  Action Port : ActionPort
  Constant : Constant  Value=DMPGCMDREACHED_CNT_U08
  Constant1 : Constant  OutDataTypeStr=uint8
      settings: AttributesFormatString=%<OutDataTypeStr>
  CopyRight2 : Subsystem  Description=|  mask(Copyright Information){none=on}
      | Copyright info block.                                               
      |                                                                     
      | Place copyright information at the top of every subsystem in design.
      mask prompts: none "No parameters"
      mask help: Place copyright information at the top of every subsystem in design.
      mask Display:
      | NxtrConf = 'Nexteer Confidential';
      | 
      | sys = bdroot; %handle for the current model ("system")
      | first = get_param(sys,'Created');
      | first = first(end-3:end);  %year is last four digits
      | 
      | last = get_param(sys,'LastModifiedDate');
      | if isempty(last)
      |     last = datestr(now,'yyyy');
      | else
      |     last = last(end-3:end);
      | end
      | 
      | if strcmp(first,last)
      |     fprintf('%s -- Copyright %s Nexteer',NxtrConf,first)
      | else
      |     fprintf('%s -- %s%s- %s Nexteer',NxtrConf,char(169),first,last)
      | end
  Product1 : Product
  Bit0Sts : Outport
  wires:
  Constant/1 -> Product1/2
  Constant1/1 -> Product1/1
  Product1/1 -> Bit0Sts/1

== system SF035A_DampgPahFwl/DampgPahFwl/DampgPahFwlPer1/Normal Firewall Operation/Set_Faults/Set NtcDmpgFwlReached/If Action Subsystem1 ==
  Action Port : ActionPort
  Constant : Constant  Value=DMPGCMDREACHED_CNT_U08
  Constant1 : Constant  Value=0  OutDataTypeStr=uint8
      settings: AttributesFormatString=%<OutDataTypeStr>
  CopyRight2 : Subsystem  Description=|  mask(Copyright Information){none=on}
      | Copyright info block.                                               
      |                                                                     
      | Place copyright information at the top of every subsystem in design.
      mask prompts: none "No parameters"
      mask help: Place copyright information at the top of every subsystem in design.
      mask Display:
      | NxtrConf = 'Nexteer Confidential';
      | 
      | sys = bdroot; %handle for the current model ("system")
      | first = get_param(sys,'Created');
      | first = first(end-3:end);  %year is last four digits
      | 
      | last = get_param(sys,'LastModifiedDate');
      | if isempty(last)
      |     last = datestr(now,'yyyy');
      | else
      |     last = last(end-3:end);
      | end
      | 
      | if strcmp(first,last)
      |     fprintf('%s -- Copyright %s Nexteer',NxtrConf,first)
      | else
      |     fprintf('%s -- %s%s- %s Nexteer',NxtrConf,char(169),first,last)
      | end
  Product1 : Product
  Bit0Sts : Outport
  wires:
  Constant/1 -> Product1/2
  Constant1/1 -> Product1/1
  Product1/1 -> Bit0Sts/1

== system SF035A_DampgPahFwl/DampgPahFwl/DampgPahFwlPer1/Normal Firewall Operation/Set_Faults/Set NtcDmpgFwlReached/If Action Subsystem2 ==
  Action Port : ActionPort
  Constant1 : Constant  OutDataTypeStr=uint8
      settings: AttributesFormatString=%<OutDataTypeStr>
  Constant2 : Constant  Value=VBICCMDREACHED_CNT_U08
  CopyRight2 : Subsystem  Description=|  mask(Copyright Information){none=on}
      | Copyright info block.                                               
      |                                                                     
      | Place copyright information at the top of every subsystem in design.
      mask prompts: none "No parameters"
      mask help: Place copyright information at the top of every subsystem in design.
      mask Display:
      | NxtrConf = 'Nexteer Confidential';
      | 
      | sys = bdroot; %handle for the current model ("system")
      | first = get_param(sys,'Created');
      | first = first(end-3:end);  %year is last four digits
      | 
      | last = get_param(sys,'LastModifiedDate');
      | if isempty(last)
      |     last = datestr(now,'yyyy');
      | else
      |     last = last(end-3:end);
      | end
      | 
      | if strcmp(first,last)
      |     fprintf('%s -- Copyright %s Nexteer',NxtrConf,first)
      | else
      |     fprintf('%s -- %s%s- %s Nexteer',NxtrConf,char(169),first,last)
      | end
  Product2 : Product
  Bit1Sts : Outport
  wires:
  Constant1/1 -> Product2/1
  Constant2/1 -> Product2/2
  Product2/1 -> Bit1Sts/1

== system SF035A_DampgPahFwl/DampgPahFwl/DampgPahFwlPer1/Normal Firewall Operation/Set_Faults/Set NtcDmpgFwlReached/If Action Subsystem3 ==
  Action Port : ActionPort
  Constant1 : Constant  Value=0  OutDataTypeStr=uint8
      settings: AttributesFormatString=%<OutDataTypeStr>
  Constant2 : Constant  Value=VBICCMDREACHED_CNT_U08
  CopyRight2 : Subsystem  Description=|  mask(Copyright Information){none=on}
      | Copyright info block.                                               
      |                                                                     
      | Place copyright information at the top of every subsystem in design.
      mask prompts: none "No parameters"
      mask help: Place copyright information at the top of every subsystem in design.
      mask Display:
      | NxtrConf = 'Nexteer Confidential';
      | 
      | sys = bdroot; %handle for the current model ("system")
      | first = get_param(sys,'Created');
      | first = first(end-3:end);  %year is last four digits
      | 
      | last = get_param(sys,'LastModifiedDate');
      | if isempty(last)
      |     last = datestr(now,'yyyy');
      | else
      |     last = last(end-3:end);
      | end
      | 
      | if strcmp(first,last)
      |     fprintf('%s -- Copyright %s Nexteer',NxtrConf,first)
      | else
      |     fprintf('%s -- %s%s- %s Nexteer',NxtrConf,char(169),first,last)
      | end
  Product2 : Product
  Bit1Sts : Outport
  wires:
  Product2/1 -> Bit1Sts/1
  Constant1/1 -> Product2/1
  Constant2/1 -> Product2/2
